simulink library "SUB_L4_Task_10ms_SUB_STATE_CONTROL"  (R2018a)
settings: Solver=VariableStepAuto  StartTime=0.0  StopTime=10.0  RelTol=1e-3
undefined symbols (not defined in the file or in its folder): ENUM_J1939_SWITCH_T, magnitude
libraries: EmE_MBD_Blockset x24, PTC_MBDS_LIB x5, simulink x5
settings Model: Creator=Chris.Balton  LastModifiedBy=Gavin.Coelho

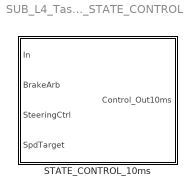
== system SUB_L4_Task_10ms_SUB_STATE_CONTROL ==
  STATE_CONTROL_10ms : Subsystem

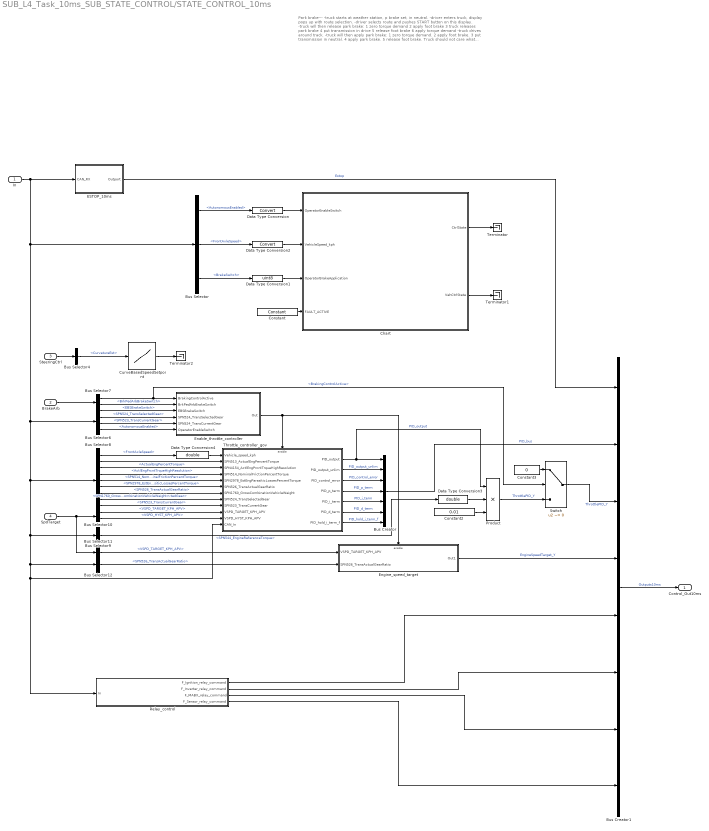
== system SUB_L4_Task_10ms_SUB_STATE_CONTROL/STATE_CONTROL_10ms ==
  note: Park brake---
      |
      |
      | -truck starts at weather station, p brake set, in neutral.
      | -driver enters truck, display pops up with route selection.
      | -driver selects route and pushes START button on this display.
      |
      | -truck will then release park brake:
      | 	1 zero torque demand
      | 	2 apply foot brake
      | 	3 truck releases park brake
      | 	4 put transmission in drive
      | 	5 release foot brake
      | 	6 apply torque demand
      |
      | -truck drives around track.
      |
      | -truck will then apply park brake:
      |
      | 	1 zero torque demand.
      | 	2 apply foot brake.
      | 	3 put transmission in neutral.
      | 	4 apply park brake.
      | 	5 release foot brake.
      |
      | Truck should not care what position the driver demanded transmission selector is in (stalk
      | position)
  In : Inport
  BrakeArb : Inport  Port=2
  SteeringCtrl : Inport  Port=3
  SpdTarget : Inport  Port=4
  Bus Creator : BusCreator  Inputs=7
  Bus Creator1 : BusCreator  Inputs=8
  Bus Selector : BusSelector  OutputSignals=DIO_Bus.AutonomousEnabled,CAN.EBC2_0B.FrontAxleSpeed,CAN.CCVS_31.BrakeSwitch
  Bus Selector10 : BusSelector  OutputSignals=VSPD_TARGET_KPH_APV,VSPD_HYST_KPH_APV
  Bus Selector11 : BusSelector  OutputSignals=VSPD_TARGET_KPH_APV
  Bus Selector12 : BusSelector  OutputSignals=CAN.ETC2_03.SPN526_TransActualGearRatio
  Bus Selector4 : BusSelector  OutputSignals=CurvatureEst
  Bus Selector6 : BusSelector  OutputSignals=CAN.EBC1_0B.EBSBrakeSwitch,CAN.ETC2_03.SPN524_TransSelectedGear,CAN.ETC2_03.SPN523_TransCurrentGear,AutonomousState.AutonomousEnabled
  Bus Selector7 : BusSelector  OutputSignals=BrakingControlActive,BrkPedArbBrakeSwitch
  Bus Selector8 : BusSelector  OutputSignals=CAN.EBC2_0B.FrontAxleSpeed,CAN.EEC1_00.ActualEngPercentTorque,CAN.EEC1_00.ActlEngPrcntTrqueHighResolution,CAN.EEC3_00.SPN514_NominalFrictionPercentTorque,CAN.EEC3_00.SPN2978_EstEngParasiticLossesPercentTorque,CAN.ETC2_03.SPN526_TransActualGearRatio,CAN.CVW_0B.SPN1760_GrossCombinationVehicleWeight,CAN.ETC2_03.SPN524_TransSelectedGear,CAN.ETC2_03.SPN523_TransCurrentGear
  Bus Selector9 : BusSelector  OutputSignals=CAN.EC1_00.SPN544_EngineReferenceTorque
  Chart : Stateflow chart  TreatAsAtomicUnit=on
      settings: CopyFcn=|
      | if strcmp(get(gcbh, 'LinkStatus'), 'resolved')
      |     set(gcbh, 'LinkStatus', 'none');
      | end
  Constant : PTC_MBDS_LIB/Extras/Sources/Constant  Value2=false  PTC_MBDS_BlockVersion=5.41  PTC_BlockType=PTC_MBDS_Constant
      settings: SourceProductName=PACCAR Technical Center MBDS Library
  Constant2 : Constant  Value=0.01
  Constant3 : Constant  Value=0
  CurveBasedSpeedSetpoint : Lookup_n-D  NumberOfTableDimensions=1  BreakpointsForDimension1=[-.25,-.1 0 .1 .25]  Table=[25 30 35 30 25]  ExtrapMethod=Clip  UseLastTableValue=on  InputSameDT=on
      settings: AttributesFormatString=|
      | X: %<BreakpointsForDimension1>
      | Y: %<Table>
  Data Type Conversion4 : DataTypeConversion  OutDataTypeStr=double  SaturateOnIntegerOverflow=on
  Data Type Conversion : DataTypeConversion
  Data Type Conversion1 : DataTypeConversion  OutDataTypeStr=uint8
  Data Type Conversion2 : DataTypeConversion
  Data Type Conversion3 : DataTypeConversion  OutDataTypeStr=double
  ESTOP_10ms : Subsystem
  Enable_throttle_controller : Subsystem
  Engine_speed_target : Subsystem  TreatAsAtomicUnit=on
  Product : Product  Inputs=3  InputSameDT=on
  Relay_control : Subsystem
  Switch : Switch  Criteria=u2 ~= 0
  Terminator : Terminator
      settings: InitFcn=|
      | try
      |    MBDS_BlockCallback('Update', gcb);
      | end
  Terminator1 : Terminator
      settings: InitFcn=|
      | try
      |    MBDS_BlockCallback('Update', gcb);
      | end
  Terminator2 : Terminator
      settings: InitFcn=|
      | try
      |    MBDS_BlockCallback('Update', gcb);
      | end
  Throttle_controller_gov : Subsystem  TreatAsAtomicUnit=on
  Control_Out10ms : Outport
  wires:
  Relay_control/4(F_Sensor_relay_command) -> Bus Creator1/8
  Relay_control/1(F_Ignition_relay_command) -> Bus Creator1/5
  Relay_control/3(F_MABX_relay_command) -> Bus Creator1/7
  Relay_control/2(F_Inverter_relay_command) -> Bus Creator1/6
  Data Type Conversion3/1 -> Product/2
  Bus Selector12/1 -> Engine_speed_target/2(SPN526_TransActualGearRatio)  "<SPN526_TransActualGearRatio>"
  Engine_speed_target/1(Out1) -> Bus Creator1/4  "EngineSpeedTarget_Y"
  Bus Selector11/1 -> Engine_speed_target/1(VSPD_TARGET_KPH_APV)  "<VSPD_TARGET_KPH_APV>"
  Bus Selector/1 -> Data Type Conversion/1  "<AutonomousEnabled>"
  Bus Selector/2 -> Data Type Conversion2/1  "<FrontAxleSpeed>"
  Bus Selector/3 -> Data Type Conversion1/1  "<BrakeSwitch>"
  Chart/1(CtrlState) -> Terminator/1
  Chart/2(VehCtrlState) -> Terminator1/1
  Bus Creator1/1 -> Control_Out10ms/1  "Outputs10ms"
  ESTOP_10ms/1(Outport) -> Bus Creator1/1  "Estop"
  Data Type Conversion/1 -> Chart/1(OperatorEnableSwitch)
  BrakeArb/1 -> Bus Selector7/1
  SteeringCtrl/1 -> Bus Selector4/1
  Bus Selector4/1 -> CurveBasedSpeedSetpoint/1  "<CurvatureEst>"
  Data Type Conversion1/1 -> Chart/3(OperatorBrakeApplication)
  Data Type Conversion2/1 -> Chart/2(VehicleSpeed_kph)
  Switch/1 -> Bus Creator1/3  "ThrottlePID_Y"
  Bus Selector6/4 -> Enable_throttle_controller/6(OperatorEnableSwitch)  "<AutonomousEnabled>"
  Bus Selector6/3 -> Enable_throttle_controller/5(SPN524_TransCurrentGear)  "<SPN523_TransCurrentGear>"
  Bus Selector6/2 -> Enable_throttle_controller/4(SPN524_TransSelectedGear)  "<SPN524_TransSelectedGear>"
  Bus Selector6/1 -> Enable_throttle_controller/3(EBSBrakeSwitch)  "<EBSBrakeSwitch>"
  Bus Selector7/2 -> Enable_throttle_controller/2(BrkPedArbBrakeSwitch)  "<BrkPedArbBrakeSwitch>"
  Bus Selector7/1 -> Switch/2, Enable_throttle_controller/1(BrakingControlActive)  "<BrakingControlActive>"
  Enable_throttle_controller/1(Out) -> Engine_speed_target/Enable, Throttle_controller_gov/Enable
  Bus Selector8/1 -> Data Type Conversion4/1  "<FrontAxleSpeed>"
  Bus Selector8/9 -> Throttle_controller_gov/9(SPN523_TransCurrentGear)  "<SPN523_TransCurrentGear>"
  Bus Selector8/8 -> Throttle_controller_gov/8(SPN524_TransSelectedGear)  "<SPN524_TransSelectedGear>"
  Bus Selector8/2 -> Throttle_controller_gov/2(SPN513_ActualEngPercentTorque)  "<ActualEngPercentTorque>"
  Bus Selector8/3 -> Throttle_controller_gov/3(SPN4154_ActlEngPrcntTrqueHighResolution)  "<ActlEngPrcntTrqueHighResolution>"
  Bus Selector8/4 -> Throttle_controller_gov/4(SPN514_NominalFrictionPercentTorque)  "<SPN514_NominalFrictionPercentTorque>"
  Bus Selector8/5 -> Throttle_controller_gov/5(SPN2978_EstEngParasiticLossesPercentTorque)  "<SPN2978_EstEngParasiticLossesPercentTorque>"
  Bus Selector8/6 -> Throttle_controller_gov/6(SPN526_TransActualGearRatio)  "<SPN526_TransActualGearRatio>"
  Bus Selector8/7 -> Throttle_controller_gov/7(SPN1760_GrossCombinationVehicleWeight)  "<SPN1760_GrossCombinationVehicleWeight>"
  In/1 -> ESTOP_10ms/1(CAN_RX), Bus Selector/1, Throttle_controller_gov/12(CAN_In), Relay_control/1(In), Bus Selector12/1, Bus Selector9/1, Bus Selector8/1, Bus Selector6/1
  Bus Selector9/1 -> Data Type Conversion3/1  "<SPN544_EngineReferenceTorque>"
  Constant2/1 -> Product/3
  SpdTarget/1 -> Bus Selector10/1, Bus Selector11/1
  Bus Selector10/2 -> Throttle_controller_gov/11(VSPD_HYST_KPH_APV)  "<VSPD_HYST_KPH_APV>"
  Bus Selector10/1 -> Throttle_controller_gov/10(VSPD_TARGET_KPH_APV)  "<VSPD_TARGET_KPH_APV>"
  Data Type Conversion4/1 -> Throttle_controller_gov/1(Vehicle_speed_kph)
  CurveBasedSpeedSetpoint/1 -> Terminator2/1
  Throttle_controller_gov/1(PID_output) -> Product/1, Bus Creator/1  "PID_output"
  Throttle_controller_gov/7(PID_hold_i_term_f) -> Bus Creator/7  "PID_hold_i_term_f"
  Throttle_controller_gov/6(PID_d_term) -> Bus Creator/6  "PID_d_term"
  Throttle_controller_gov/5(PID_i_term) -> Bus Creator/5  "PID_i_term"
  Throttle_controller_gov/4(PID_p_term) -> Bus Creator/4  "PID_p_term"
  Throttle_controller_gov/3(PID_control_error) -> Bus Creator/3  "PID_control_error"
  Throttle_controller_gov/2(PID_output_unlim) -> Bus Creator/2  "PID_output_unlim"
  Bus Creator/1 -> Bus Creator1/2  "PID_bus"
  Product/1 -> Switch/3  "ThrottlePID_Y"
  Constant3/1 -> Switch/1
  Constant/1 -> Chart/4(FAULT_ACTIVE)

== system SUB_L4_Task_10ms_SUB_STATE_CONTROL/STATE_CONTROL_10ms/ESTOP_10ms ==
  CAN_RX : Inport
  Bus Creator : BusCreator  Inputs=1
  Constant : PTC_MBDS_LIB/Extras/Sources/Constant  Value2=false  PTC_MBDS_BlockVersion=5.41  PTC_BlockType=PTC_MBDS_Constant
      settings: SourceProductName=PACCAR Technical Center MBDS Library
  Terminator1 : Terminator
  Outport : Outport
  wires:
  Constant/1 -> Bus Creator/1
  CAN_RX/1 -> Terminator1/1
  Bus Creator/1 -> Outport/1  "Estop"

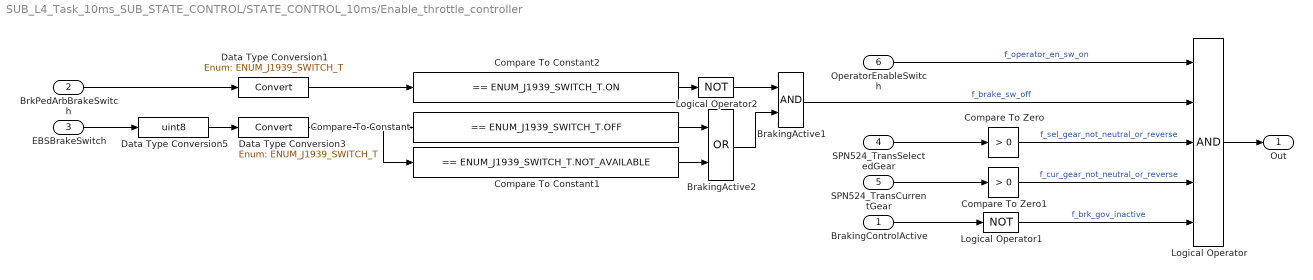
== system SUB_L4_Task_10ms_SUB_STATE_CONTROL/STATE_CONTROL_10ms/Enable_throttle_controller ==
  BrakingControlActive : Inport
  BrkPedArbBrakeSwitch : Inport  Port=2
  EBSBrakeSwitch : Inport  Port=3
  SPN524_TransSelectedGear : Inport  Port=4
  SPN524_TransCurrentGear : Inport  Port=5
  OperatorEnableSwitch : Inport  Port=6
  BrakingActive1 : Logic  OutDataTypeStr=boolean
  BrakingActive2 : Logic  Operator=OR  OutDataTypeStr=boolean
  Compare To Constant : simulink/Logic and Bit Operations/Compare To Constant  relop===  const=ENUM_J1939_SWITCH_T.OFF  OutDataTypeStr=boolean
  Compare To Constant1 : simulink/Logic and Bit Operations/Compare To Constant  relop===  const=ENUM_J1939_SWITCH_T.NOT_AVAILABLE  OutDataTypeStr=boolean
  Compare To Constant2 : simulink/Logic and Bit Operations/Compare To Constant  relop===  const=ENUM_J1939_SWITCH_T.ON  OutDataTypeStr=boolean
  Compare To Zero : simulink/Logic and Bit Operations/Compare To Zero  relop=>  OutDataTypeStr=boolean
  Compare To Zero1 : simulink/Logic and Bit Operations/Compare To Zero  relop=>  OutDataTypeStr=boolean
  Data Type Conversion1 : DataTypeConversion  OutDataTypeStr=Enum: ENUM_J1939_SWITCH_T
      settings: AttributesFormatString=%<OutDataTypeStr>
  Data Type Conversion3 : DataTypeConversion  OutDataTypeStr=Enum: ENUM_J1939_SWITCH_T
      settings: AttributesFormatString=%<OutDataTypeStr>
  Data Type Conversion5 : DataTypeConversion  OutDataTypeStr=uint8
      settings: AttributesFormatString=%<OutDataTypeStr>
  Logical Operator : Logic  Inputs=5  OutDataTypeStr=boolean
  Logical Operator1 : Logic  Operator=NOT  Inputs=4  OutDataTypeStr=boolean
  Logical Operator2 : Logic  Operator=NOT  Inputs=4  OutDataTypeStr=boolean
  Out : Outport
  wires:
  SPN524_TransSelectedGear/1 -> Compare To Zero/1
  SPN524_TransCurrentGear/1 -> Compare To Zero1/1
  BrakingControlActive/1 -> Logical Operator1/1
  Logical Operator1/1 -> Logical Operator/5  "f_brk_gov_inactive"
  Compare To Zero1/1 -> Logical Operator/4  "f_cur_gear_not_neutral_or_reverse"
  Compare To Zero/1 -> Logical Operator/3  "f_sel_gear_not_neutral_or_reverse"
  Logical Operator/1 -> Out/1
  OperatorEnableSwitch/1 -> Logical Operator/1  "f_operator_en_sw_on"
  BrakingActive1/1 -> Logical Operator/2  "f_brake_sw_off"
  EBSBrakeSwitch/1 -> Data Type Conversion5/1
  BrkPedArbBrakeSwitch/1 -> Data Type Conversion1/1
  Logical Operator2/1 -> BrakingActive1/1
  Compare To Constant/1 -> BrakingActive2/1
  Compare To Constant1/1 -> BrakingActive2/2
  BrakingActive2/1 -> BrakingActive1/2
  Data Type Conversion3/1 -> Compare To Constant/1, Compare To Constant1/1
  Data Type Conversion1/1 -> Compare To Constant2/1
  Compare To Constant2/1 -> Logical Operator2/1
  Data Type Conversion5/1 -> Data Type Conversion3/1

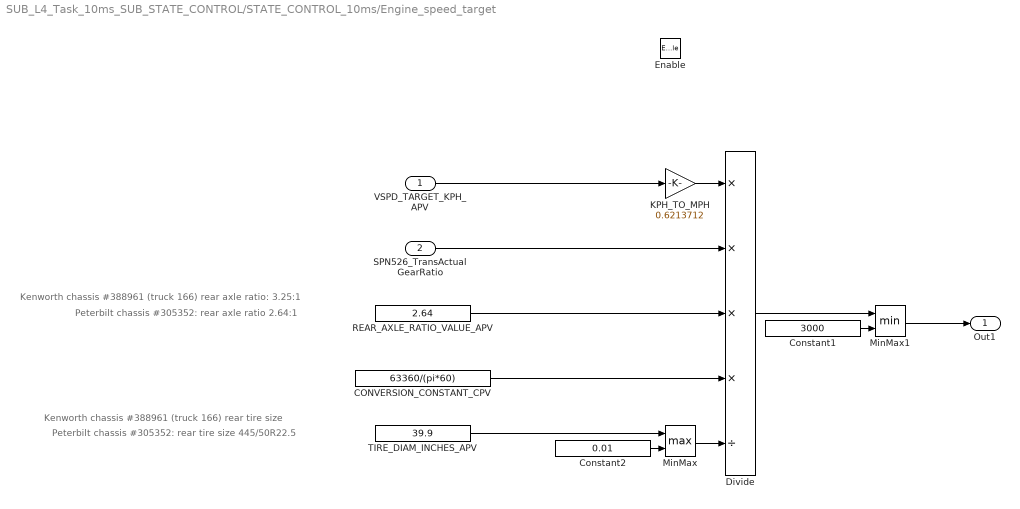
== system SUB_L4_Task_10ms_SUB_STATE_CONTROL/STATE_CONTROL_10ms/Engine_speed_target ==
  note: Kenworth chassis #388961 (truck 166) rear tire size
  note: Kenworth chassis #388961 (truck 166) rear axle ratio: 3.25:1
  note: Peterbilt chassis #305352: rear axle ratio 2.64:1
  note: Peterbilt chassis #305352: rear tire size 445/50R22.5
  VSPD_TARGET_KPH_APV : Inport
  SPN526_TransActualGearRatio : Inport  Port=2
  Enable : EnablePort  StatesWhenEnabling=reset
  CONVERSION_CONSTANT_CPV : Constant  Value=63360/(pi*60)
  Constant1 : Constant  Value=3000
  Constant2 : Constant  Value=0.01
  Divide : Product  Inputs=****/  InputSameDT=on
  KPH_TO_MPH : Gain  Gain=0.6213712  OutDataTypeStr=double
  MinMax : MinMax  Function=max  Inputs=2  InputSameDT=on
  MinMax1 : MinMax  Inputs=2  InputSameDT=on
  REAR_AXLE_RATIO_VALUE_APV : Constant  Value=2.64
  TIRE_DIAM_INCHES_APV : Constant  Value=39.9
  Out1 : Outport  OutputWhenDisabled=reset  InitialOutput=0
  wires:
  KPH_TO_MPH/1 -> Divide/1
  Constant1/1 -> MinMax1/2
  MinMax1/1 -> Out1/1
  Constant2/1 -> MinMax/2
  MinMax/1 -> Divide/5
  SPN526_TransActualGearRatio/1 -> Divide/2
  VSPD_TARGET_KPH_APV/1 -> KPH_TO_MPH/1
  REAR_AXLE_RATIO_VALUE_APV/1 -> Divide/3
  TIRE_DIAM_INCHES_APV/1 -> MinMax/1
  CONVERSION_CONSTANT_CPV/1 -> Divide/4
  Divide/1 -> MinMax1/1

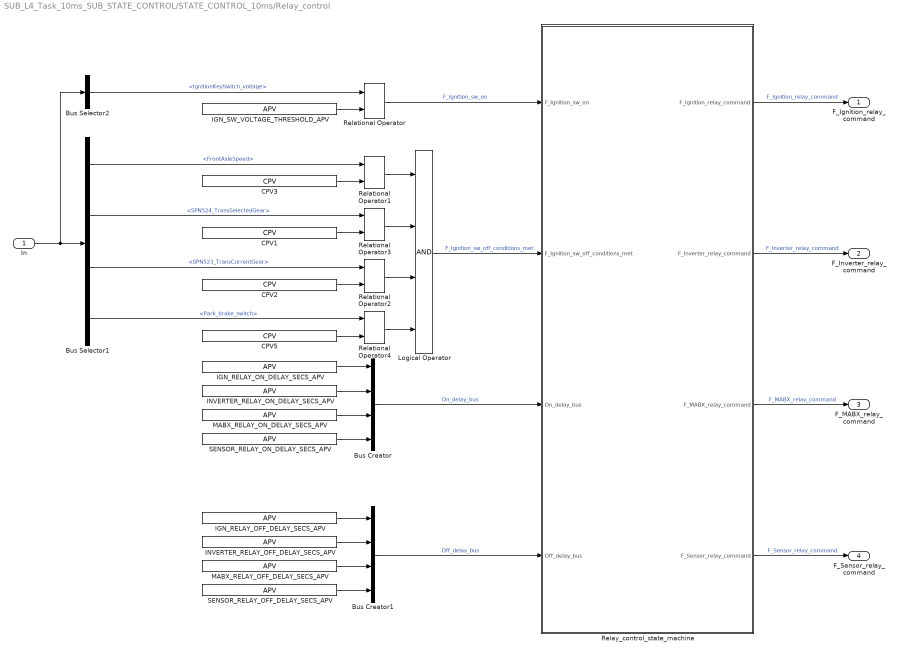
== system SUB_L4_Task_10ms_SUB_STATE_CONTROL/STATE_CONTROL_10ms/Relay_control ==
  In : Inport
  Bus Creator : BusCreator  Inputs=4
  Bus Creator1 : BusCreator  Inputs=4
  Bus Selector1 : BusSelector  OutputSignals=CAN.EBC2_0B.FrontAxleSpeed,CAN.ETC2_03.SPN524_TransSelectedGear,CAN.ETC2_03.SPN523_TransCurrentGear,CAN.CCVS_31.Park_brake_switch
  Bus Selector2 : BusSelector  OutputSignals=DIO_Bus.IgnitionKeySwitch_voltage
  CPV1 : EmE_MBD_Blockset/Sources/CPV  conval=0
      settings: SourceProductName=PACCAR EmE MBD Blockset
  CPV2 : EmE_MBD_Blockset/Sources/CPV  conval=0
      settings: SourceProductName=PACCAR EmE MBD Blockset
  CPV3 : EmE_MBD_Blockset/Sources/CPV  conval=0
      settings: SourceProductName=PACCAR EmE MBD Blockset
  CPV5 : EmE_MBD_Blockset/Sources/CPV  conval=1
      settings: SourceProductName=PACCAR EmE MBD Blockset
  IGN_RELAY_OFF_DELAY_SECS_APV : EmE_MBD_Blockset/Sources/APV  conval=0.2
      settings: SourceProductName=PACCAR EmE MBD Blockset
  IGN_RELAY_ON_DELAY_SECS_APV : EmE_MBD_Blockset/Sources/APV  conval=0.2
      settings: SourceProductName=PACCAR EmE MBD Blockset
  IGN_SW_VOLTAGE_THRESHOLD_APV : EmE_MBD_Blockset/Sources/APV  conval=6
      settings: SourceProductName=PACCAR EmE MBD Blockset
  INVERTER_RELAY_OFF_DELAY_SECS_APV : EmE_MBD_Blockset/Sources/APV  conval=0
      settings: SourceProductName=PACCAR EmE MBD Blockset
  INVERTER_RELAY_ON_DELAY_SECS_APV : EmE_MBD_Blockset/Sources/APV  conval=0
      settings: SourceProductName=PACCAR EmE MBD Blockset
  Logical Operator : Logic  Inputs=4  OutDataTypeStr=boolean
  MABX_RELAY_OFF_DELAY_SECS_APV : EmE_MBD_Blockset/Sources/APV  conval=0
      settings: SourceProductName=PACCAR EmE MBD Blockset
  MABX_RELAY_ON_DELAY_SECS_APV : EmE_MBD_Blockset/Sources/APV  conval=0
      settings: SourceProductName=PACCAR EmE MBD Blockset
  Relational Operator : EmE_MBD_Blockset/Logic and Bit Operations/Relational Operator  func=>=
      settings: SourceProductName=PACCAR EmE MBD Blockset
  Relational Operator1 : EmE_MBD_Blockset/Logic and Bit Operations/Relational Operator  func=<=
      settings: SourceProductName=PACCAR EmE MBD Blockset
  Relational Operator2 : EmE_MBD_Blockset/Logic and Bit Operations/Relational Operator  func===
      settings: SourceProductName=PACCAR EmE MBD Blockset
  Relational Operator3 : EmE_MBD_Blockset/Logic and Bit Operations/Relational Operator  func===
      settings: SourceProductName=PACCAR EmE MBD Blockset
  Relational Operator4 : EmE_MBD_Blockset/Logic and Bit Operations/Relational Operator  func===
      settings: SourceProductName=PACCAR EmE MBD Blockset
  Relay_control_state_machine : Stateflow chart  TreatAsAtomicUnit=on
  SENSOR_RELAY_OFF_DELAY_SECS_APV : EmE_MBD_Blockset/Sources/APV  conval=0
      settings: SourceProductName=PACCAR EmE MBD Blockset
  SENSOR_RELAY_ON_DELAY_SECS_APV : EmE_MBD_Blockset/Sources/APV  conval=0
      settings: SourceProductName=PACCAR EmE MBD Blockset
  F_Ignition_relay_command : Outport
  F_Inverter_relay_command : Outport  Port=2
  F_MABX_relay_command : Outport  Port=3
  F_Sensor_relay_command : Outport  Port=4
  wires:
  Bus Selector1/1 -> Relational Operator1/1  "<FrontAxleSpeed>"
  Relay_control_state_machine/2(F_Inverter_relay_command) -> F_Inverter_relay_command/1  "F_Inverter_relay_command"
  Bus Selector1/3 -> Relational Operator2/1  "<SPN523_TransCurrentGear>"
  IGN_RELAY_ON_DELAY_SECS_APV/1 -> Bus Creator/1
  Bus Selector2/1 -> Relational Operator/1  "<IgnitionKeySwitch_voltage>"
  Bus Selector1/2 -> Relational Operator3/1  "<SPN524_TransSelectedGear>"
  Relay_control_state_machine/1(F_Ignition_relay_command) -> F_Ignition_relay_command/1  "F_Ignition_relay_command"
  Bus Selector1/4 -> Relational Operator4/1  "<Park_brake_switch>"
  Relay_control_state_machine/3(F_MABX_relay_command) -> F_MABX_relay_command/1  "F_MABX_relay_command"
  Relay_control_state_machine/4(F_Sensor_relay_command) -> F_Sensor_relay_command/1  "F_Sensor_relay_command"
  Relational Operator3/1 -> Logical Operator/2
  CPV2/1 -> Relational Operator2/2
  Relational Operator2/1 -> Logical Operator/3
  CPV1/1 -> Relational Operator3/2
  Relational Operator/1 -> Relay_control_state_machine/1(F_Ignition_sw_on)  "F_Ignition_sw_on"
  CPV3/1 -> Relational Operator1/2
  Relational Operator4/1 -> Logical Operator/4
  Relational Operator1/1 -> Logical Operator/1
  Bus Creator1/1 -> Relay_control_state_machine/4(Off_delay_bus)  "Off_delay_bus"
  INVERTER_RELAY_ON_DELAY_SECS_APV/1 -> Bus Creator/2
  Logical Operator/1 -> Relay_control_state_machine/2(F_Ignition_sw_off_conditions_met)  "F_Ignition_sw_off_conditions_met"
  SENSOR_RELAY_ON_DELAY_SECS_APV/1 -> Bus Creator/4
  MABX_RELAY_ON_DELAY_SECS_APV/1 -> Bus Creator/3
  Bus Creator/1 -> Relay_control_state_machine/3(On_delay_bus)  "On_delay_bus"
  CPV5/1 -> Relational Operator4/2
  MABX_RELAY_OFF_DELAY_SECS_APV/1 -> Bus Creator1/3
  SENSOR_RELAY_OFF_DELAY_SECS_APV/1 -> Bus Creator1/4
  IGN_RELAY_OFF_DELAY_SECS_APV/1 -> Bus Creator1/1
  IGN_SW_VOLTAGE_THRESHOLD_APV/1 -> Relational Operator/2
  INVERTER_RELAY_OFF_DELAY_SECS_APV/1 -> Bus Creator1/2
  In/1 -> Bus Selector1/1, Bus Selector2/1

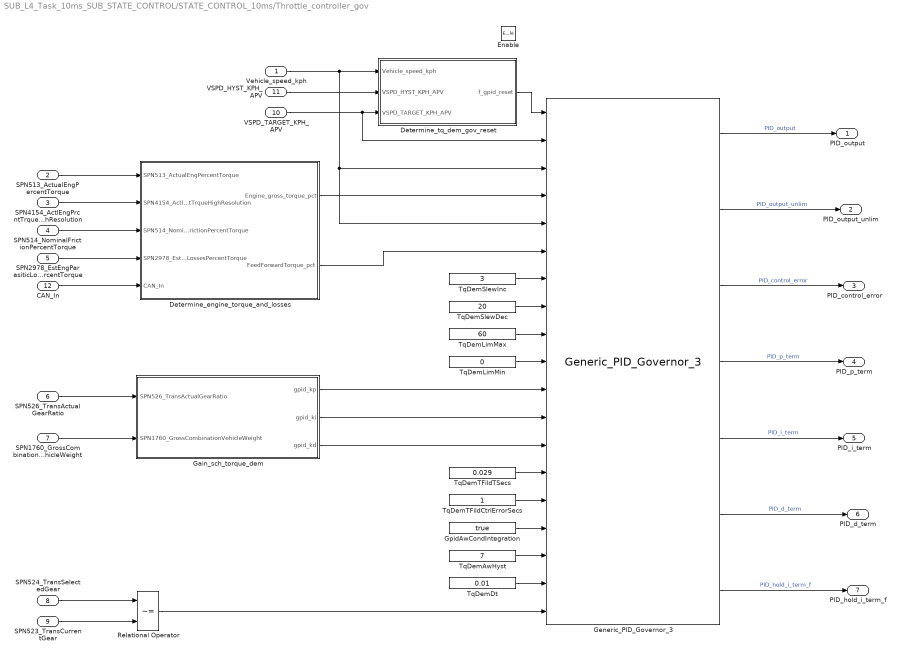
== system SUB_L4_Task_10ms_SUB_STATE_CONTROL/STATE_CONTROL_10ms/Throttle_controller_gov ==
  Vehicle_speed_kph : Inport
  SPN513_ActualEngPercentTorque : Inport  Port=2
  SPN4154_ActlEngPrcntTrqueHighResolution : Inport  Port=3
  SPN514_NominalFrictionPercentTorque : Inport  Port=4
  SPN2978_EstEngParasiticLossesPercentTorque : Inport  Port=5
  SPN526_TransActualGearRatio : Inport  Port=6
  SPN1760_GrossCombinationVehicleWeight : Inport  Port=7
  SPN524_TransSelectedGear : Inport  Port=8
  SPN523_TransCurrentGear : Inport  Port=9
  VSPD_TARGET_KPH_APV : Inport  Port=10
  VSPD_HYST_KPH_APV : Inport  Port=11
  CAN_In : Inport  Port=12
  Enable : EnablePort  StatesWhenEnabling=reset
  Determine_engine_torque_and_losses : Subsystem
  Determine_tq_dem_gov_reset : Subsystem
  Gain_sch_torque_dem : Subsystem
  Generic_PID_Governor_3 : EmE_MBD_Blockset/Controllers/Generic_PID_Governor_3
      settings: SourceProductName=PACCAR EmE MBD Blockset
  GpidAwCondIntegration : Constant  Value=true
  Relational Operator : RelationalOperator  Operator=~=  OutDataTypeStr=boolean  RndMeth=Nearest  InputSameDT=on
  TqDemAwHyst : Constant  Value=7
  TqDemDt : Constant  Value=0.01
  TqDemLimMax : Constant  Value=60
  TqDemLimMin : Constant  Value=0
  TqDemSlewDec : Constant  Value=20
  TqDemSlewInc : Constant  Value=3
  TqDemTFildCtrlErrorSecs : Constant
  TqDemTFildTSecs : Constant  Value=0.029
  PID_output : Outport  OutputWhenDisabled=reset  InitialOutput=0
  PID_output_unlim : Outport  Port=2  OutputWhenDisabled=reset  InitialOutput=0
  PID_control_error : Outport  Port=3  OutputWhenDisabled=reset  InitialOutput=0
  PID_p_term : Outport  Port=4  OutputWhenDisabled=reset  InitialOutput=0
  PID_i_term : Outport  Port=5  OutputWhenDisabled=reset  InitialOutput=0
  PID_d_term : Outport  Port=6  OutputWhenDisabled=reset  InitialOutput=0
  PID_hold_i_term_f : Outport  Port=7  OutputWhenDisabled=reset  InitialOutput=false
  wires:
  Vehicle_speed_kph/1 -> Generic_PID_Governor_3/5, Generic_PID_Governor_3/3, Determine_tq_dem_gov_reset/1(Vehicle_speed_kph)
  VSPD_HYST_KPH_APV/1 -> Determine_tq_dem_gov_reset/2(VSPD_HYST_KPH_APV)
  SPN513_ActualEngPercentTorque/1 -> Determine_engine_torque_and_losses/1(SPN513_ActualEngPercentTorque)
  SPN4154_ActlEngPrcntTrqueHighResolution/1 -> Determine_engine_torque_and_losses/2(SPN4154_ActlEngPrcntTrqueHighResolution)
  SPN514_NominalFrictionPercentTorque/1 -> Determine_engine_torque_and_losses/3(SPN514_NominalFrictionPercentTorque)
  SPN2978_EstEngParasiticLossesPercentTorque/1 -> Determine_engine_torque_and_losses/4(SPN2978_EstEngParasiticLossesPercentTorque)
  SPN526_TransActualGearRatio/1 -> Gain_sch_torque_dem/1(SPN526_TransActualGearRatio)
  SPN1760_GrossCombinationVehicleWeight/1 -> Gain_sch_torque_dem/2(SPN1760_GrossCombinationVehicleWeight)
  SPN523_TransCurrentGear/1 -> Relational Operator/2
  SPN524_TransSelectedGear/1 -> Relational Operator/1
  Determine_tq_dem_gov_reset/1(f_gpid_reset) -> Generic_PID_Governor_3/1
  Determine_engine_torque_and_losses/1(Engine_gross_torque_pct) -> Generic_PID_Governor_3/4
  Determine_engine_torque_and_losses/2(FeedForwardTorque_pct) -> Generic_PID_Governor_3/6
  Relational Operator/1 -> Generic_PID_Governor_3/19
  Gain_sch_torque_dem/1(gpid_kp) -> Generic_PID_Governor_3/11
  Gain_sch_torque_dem/2(gpid_ki) -> Generic_PID_Governor_3/12
  Gain_sch_torque_dem/3(gpid_kd) -> Generic_PID_Governor_3/13
  TqDemLimMin/1 -> Generic_PID_Governor_3/10
  TqDemLimMax/1 -> Generic_PID_Governor_3/9
  TqDemSlewInc/1 -> Generic_PID_Governor_3/7
  TqDemSlewDec/1 -> Generic_PID_Governor_3/8
  TqDemTFildTSecs/1 -> Generic_PID_Governor_3/14
  TqDemTFildCtrlErrorSecs/1 -> Generic_PID_Governor_3/15
  GpidAwCondIntegration/1 -> Generic_PID_Governor_3/16
  TqDemAwHyst/1 -> Generic_PID_Governor_3/17
  TqDemDt/1 -> Generic_PID_Governor_3/18
  Generic_PID_Governor_3/2 -> PID_output_unlim/1  "PID_output_unlim"
  Generic_PID_Governor_3/1 -> PID_output/1  "PID_output"
  Generic_PID_Governor_3/3 -> PID_control_error/1  "PID_control_error"
  Generic_PID_Governor_3/4 -> PID_p_term/1  "PID_p_term"
  Generic_PID_Governor_3/5 -> PID_i_term/1  "PID_i_term"
  Generic_PID_Governor_3/6 -> PID_d_term/1  "PID_d_term"
  Generic_PID_Governor_3/7 -> PID_hold_i_term_f/1  "PID_hold_i_term_f"
  VSPD_TARGET_KPH_APV/1 -> Generic_PID_Governor_3/2, Determine_tq_dem_gov_reset/3(VSPD_TARGET_KPH_APV)
  CAN_In/1 -> Determine_engine_torque_and_losses/5(CAN_In)

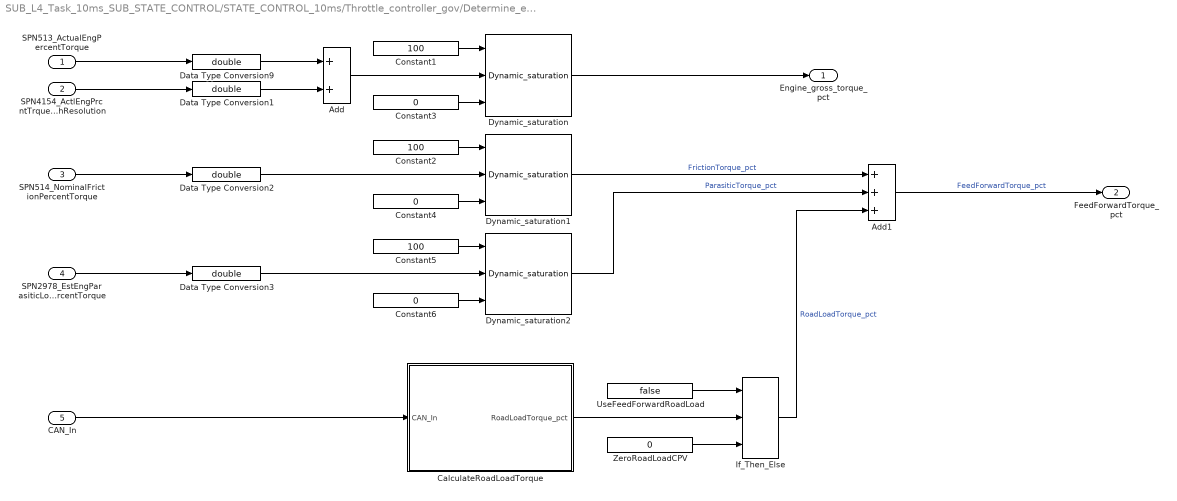
== system SUB_L4_Task_10ms_SUB_STATE_CONTROL/STATE_CONTROL_10ms/Throttle_controller_gov/Determine_engine_torque_and_losses ==
  SPN513_ActualEngPercentTorque : Inport
  SPN4154_ActlEngPrcntTrqueHighResolution : Inport  Port=2
  SPN514_NominalFrictionPercentTorque : Inport  Port=3
  SPN2978_EstEngParasiticLossesPercentTorque : Inport  Port=4
  CAN_In : Inport  Port=5
  Add : Sum  InputSameDT=on
  Add1 : Sum  Inputs=+++  InputSameDT=on
  CalculateRoadLoadTorque : Subsystem
  Constant1 : Constant  Value=100
  Constant2 : Constant  Value=100
  Constant3 : Constant  Value=0
  Constant4 : Constant  Value=0
  Constant5 : Constant  Value=100
  Constant6 : Constant  Value=0
  Data Type Conversion{1..3,9} (4 alike) : DataTypeConversion  OutDataTypeStr=double  SaturateOnIntegerOverflow=on
  Dynamic_saturation : EmE_MBD_Blockset/Discontinuities/Dynamic_saturation
      settings: SourceProductName=PACCAR EmE MBD Blockset
  Dynamic_saturation1 : EmE_MBD_Blockset/Discontinuities/Dynamic_saturation
      settings: SourceProductName=PACCAR EmE MBD Blockset
  Dynamic_saturation2 : EmE_MBD_Blockset/Discontinuities/Dynamic_saturation
      settings: SourceProductName=PACCAR EmE MBD Blockset
  If_Then_Else : EmE_MBD_Blockset/Signal Routing/If_Then_Else
      settings: SourceProductName=PACCAR EmE MBD Blockset
  UseFeedForwardRoadLoad : Constant  Value=false  OutDataTypeStr=boolean
  ZeroRoadLoadCPV : Constant  Value=0
  Engine_gross_torque_pct : Outport
  FeedForwardTorque_pct : Outport  Port=2
  wires:
  SPN513_ActualEngPercentTorque/1 -> Data Type Conversion9/1
  SPN4154_ActlEngPrcntTrqueHighResolution/1 -> Data Type Conversion1/1
  Add/1 -> Dynamic_saturation/2
  Constant3/1 -> Dynamic_saturation/3
  Constant1/1 -> Dynamic_saturation/1
  SPN514_NominalFrictionPercentTorque/1 -> Data Type Conversion2/1
  Constant4/1 -> Dynamic_saturation1/3
  Constant2/1 -> Dynamic_saturation1/1
  SPN2978_EstEngParasiticLossesPercentTorque/1 -> Data Type Conversion3/1
  Constant6/1 -> Dynamic_saturation2/3
  Constant5/1 -> Dynamic_saturation2/1
  Dynamic_saturation1/1 -> Add1/1  "FrictionTorque_pct"
  Dynamic_saturation2/1 -> Add1/2  "ParasiticTorque_pct"
  Dynamic_saturation/1 -> Engine_gross_torque_pct/1
  Add1/1 -> FeedForwardTorque_pct/1  "FeedForwardTorque_pct"
  Data Type Conversion9/1 -> Add/1
  Data Type Conversion1/1 -> Add/2
  Data Type Conversion2/1 -> Dynamic_saturation1/2
  Data Type Conversion3/1 -> Dynamic_saturation2/2
  CAN_In/1 -> CalculateRoadLoadTorque/1(CAN_In)
  CalculateRoadLoadTorque/1(RoadLoadTorque_pct) -> If_Then_Else/2
  If_Then_Else/1 -> Add1/3  "RoadLoadTorque_pct"
  ZeroRoadLoadCPV/1 -> If_Then_Else/3
  UseFeedForwardRoadLoad/1 -> If_Then_Else/1

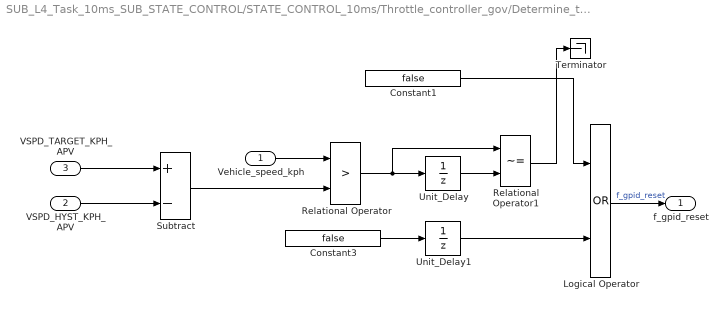
== system SUB_L4_Task_10ms_SUB_STATE_CONTROL/STATE_CONTROL_10ms/Throttle_controller_gov/Determine_tq_dem_gov_reset ==
  Vehicle_speed_kph : Inport
  VSPD_HYST_KPH_APV : Inport  Port=2
  VSPD_TARGET_KPH_APV : Inport  Port=3
  Constant1 : Constant  Value=false
  Constant3 : Constant  Value=false
  Logical Operator : Logic  Operator=OR  AllPortsSameDT=off  OutDataTypeStr=boolean
  Relational Operator : RelationalOperator  Operator=>  OutDataTypeStr=boolean  RndMeth=Nearest  InputSameDT=on
  Relational Operator1 : RelationalOperator  Operator=~=  OutDataTypeStr=boolean  RndMeth=Nearest  InputSameDT=on
  Subtract : Sum  Inputs=+-  InputSameDT=on
  Terminator : Terminator
  Unit_Delay : UnitDelay  SampleTime=-1
      settings: AttributesFormatString=IC: %<vinit>
  Unit_Delay1 : UnitDelay  InitialCondition=true  SampleTime=-1
      settings: AttributesFormatString=IC: %<vinit>
  f_gpid_reset : Outport
  wires:
  VSPD_TARGET_KPH_APV/1 -> Subtract/1
  VSPD_HYST_KPH_APV/1 -> Subtract/2
  Vehicle_speed_kph/1 -> Relational Operator/1
  Subtract/1 -> Relational Operator/2
  Relational Operator/1 -> Unit_Delay/1, Relational Operator1/1
  Unit_Delay/1 -> Relational Operator1/2
  Relational Operator1/1 -> Terminator/1
  Logical Operator/1 -> f_gpid_reset/1  "f_gpid_reset"
  Unit_Delay1/1 -> Logical Operator/2
  Constant3/1 -> Unit_Delay1/1
  Constant1/1 -> Logical Operator/1

== system SUB_L4_Task_10ms_SUB_STATE_CONTROL/STATE_CONTROL_10ms/Throttle_controller_gov/Gain_sch_torque_dem ==
  SPN526_TransActualGearRatio : Inport
  SPN1760_GrossCombinationVehicleWeight : Inport  Port=2
  2D_Lookup_Table : PTC_MBDS_LIB/Extras/Lookup Tables/2D_Lookup_Table  ParameterObjectName=TQ_DEM_KP_DATA_MPV  InterpolationMethod=Linear  PTC_MBDS_BlockVersion=5.41  PTC_BlockType=PTC_MBDS_2D_Lookup_Table
      settings: SourceProductName=PACCAR Technical Center MBDS Library
      settings: AttributesFormatString=|
      | Row Axis: TQ_DEM_MASS_STEP_MPV (kg)
      | Column Axis: TQ_DEM_GEAR_RATIO_STEP_MPV (1)
      | Data Axis: TQ_DEM_KP_DATA_MPV (1)
      | Interpolation Method: Linear
  2D_Lookup_Table1 : PTC_MBDS_LIB/Extras/Lookup Tables/2D_Lookup_Table  ParameterObjectName=TQ_DEM_KI_DATA_MPV  InterpolationMethod=Linear  PTC_MBDS_BlockVersion=5.41  PTC_BlockType=PTC_MBDS_2D_Lookup_Table
      settings: SourceProductName=PACCAR Technical Center MBDS Library
      settings: AttributesFormatString=|
      | Row Axis: TQ_DEM_MASS_STEP_MPV (kg)
      | Column Axis: TQ_DEM_GEAR_RATIO_STEP_MPV (1)
      | Data Axis: TQ_DEM_KI_DATA_MPV (1/s)
      | Interpolation Method: Linear
  2D_Lookup_Table2 : PTC_MBDS_LIB/Extras/Lookup Tables/2D_Lookup_Table  ParameterObjectName=TQ_DEM_KD_DATA_MPV  InterpolationMethod=Linear  PTC_MBDS_BlockVersion=5.41  PTC_BlockType=PTC_MBDS_2D_Lookup_Table
      settings: SourceProductName=PACCAR Technical Center MBDS Library
      settings: AttributesFormatString=|
      | Row Axis: TQ_DEM_MASS_STEP_MPV (kg)
      | Column Axis: TQ_DEM_GEAR_RATIO_STEP_MPV (1)
      | Data Axis: TQ_DEM_KD_DATA_MPV (s)
      | Interpolation Method: Linear
  gpid_kp : Outport
  gpid_ki : Outport  Port=2
  gpid_kd : Outport  Port=3
  wires:
  2D_Lookup_Table/1 -> gpid_kp/1
  SPN526_TransActualGearRatio/1 -> 2D_Lookup_Table/2, 2D_Lookup_Table2/2, 2D_Lookup_Table1/2
  SPN1760_GrossCombinationVehicleWeight/1 -> 2D_Lookup_Table/1, 2D_Lookup_Table2/1, 2D_Lookup_Table1/1
  2D_Lookup_Table1/1 -> gpid_ki/1
  2D_Lookup_Table2/1 -> gpid_kd/1

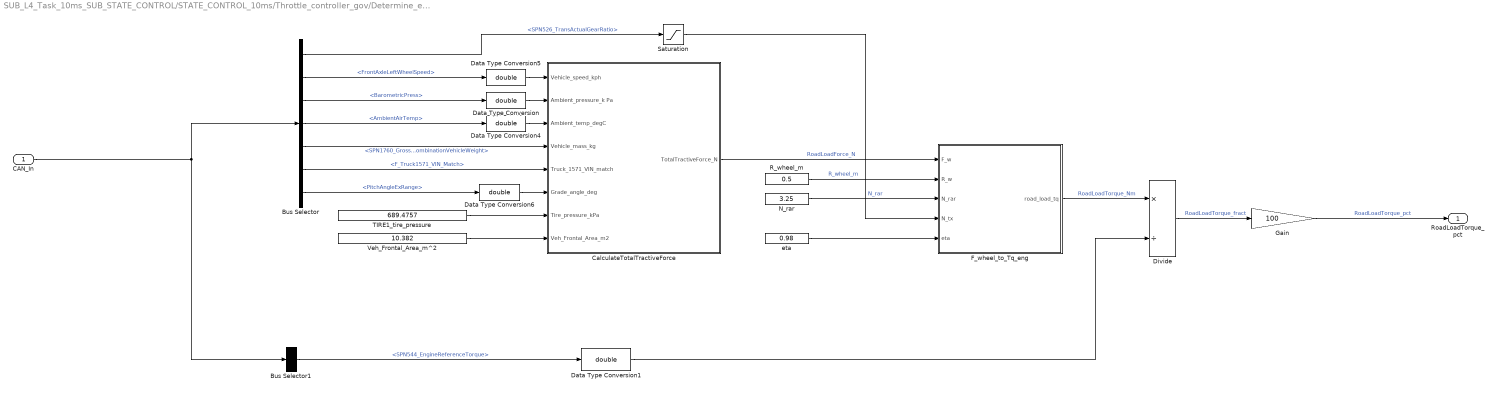
== system SUB_L4_Task_10ms_SUB_STATE_CONTROL/STATE_CONTROL_10ms/Throttle_controller_gov/Determine_engine_torque_and_losses/CalculateRoadLoadTorque ==
  CAN_In : Inport
  Bus Selector : BusSelector  OutputSignals=CAN.ETC2_03.SPN526_TransActualGearRatio,CAN.HRW_0B.FrontAxleLeftWheelSpeed,CAN.AMB_00.BarometricPress,CAN.AMB_00.AmbientAirTemp,CAN.CVW_0B.SPN1760_GrossCombinationVehicleWeight,CAN.VI_00.F_Truck1571_VIN_Match,CAN.SSI2_03.PitchAngleExRange
  Bus Selector1 : BusSelector  OutputSignals=CAN.EC1_00.SPN544_EngineReferenceTorque
  CalculateTotalTractiveForce : Subsystem
  Data Type Conversion{,1,4..6} (5 alike) : DataTypeConversion  OutDataTypeStr=double
      Data Type Conversion settings: AttributesFormatString=%<OutDataTypeStr>
      Data Type Conversion4 settings: AttributesFormatString=%<OutDataTypeStr>
      Data Type Conversion5 settings: AttributesFormatString=%<OutDataTypeStr>
      Data Type Conversion6 settings: AttributesFormatString=%<OutDataTypeStr>
  Divide : Product  Inputs=*/  InputSameDT=on
  F_wheel_to_Tq_eng : MATLAB Function  TreatAsAtomicUnit=on
  Gain : Gain  Gain=100
  N_rar : Constant  Value=3.25
  R_wheel_m : Constant  Value=0.5
  Saturation : Saturate  UpperLimit=20  LowerLimit=0.1
  TIRE1_tire_pressure : Constant  Value=689.4757
  Veh_Frontal_Area_m^2 : Constant  Value=10.382
  eta : Constant  Value=0.98
  RoadLoadTorque_pct : Outport
  wires:
  Data Type Conversion1/1 -> Divide/2
  Divide/1 -> Gain/1  "RoadLoadTorque_fract"
  CalculateTotalTractiveForce/1(TotalTractiveForce_N) -> F_wheel_to_Tq_eng/1(F_w)  "RoadLoadForce_N"
  Bus Selector/6 -> CalculateTotalTractiveForce/5(Truck_1571_VIN_match)  "<F_Truck1571_VIN_Match>"
  Bus Selector/3 -> Data Type Conversion/1  "<BarometricPress>"
  TIRE1_tire_pressure/1 -> CalculateTotalTractiveForce/7(Tire_pressure_kPa)
  Veh_Frontal_Area_m^2/1 -> CalculateTotalTractiveForce/8(Veh_Frontal_Area_m2)
  Data Type Conversion/1 -> CalculateTotalTractiveForce/2(Ambient_pressure_k Pa)
  Bus Selector/7 -> Data Type Conversion6/1  "<PitchAngleExRange>"
  Bus Selector/2 -> Data Type Conversion5/1  "<FrontAxleLeftWheelSpeed>"
  Data Type Conversion4/1 -> CalculateTotalTractiveForce/3(Ambient_temp_degC)
  Bus Selector/4 -> Data Type Conversion4/1  "<AmbientAirTemp>"
  Data Type Conversion5/1 -> CalculateTotalTractiveForce/1(Vehicle_speed_kph)
  CAN_In/1 -> Bus Selector1/1, Bus Selector/1
  Bus Selector/5 -> CalculateTotalTractiveForce/4(Vehicle_mass_kg)  "<SPN1760_GrossCombinationVehicleWeight>"
  F_wheel_to_Tq_eng/1(road_load_tq) -> Divide/1  "RoadLoadTorque_Nm"
  R_wheel_m/1 -> F_wheel_to_Tq_eng/2(R_w)  "R_wheel_m"
  eta/1 -> F_wheel_to_Tq_eng/5(eta)
  N_rar/1 -> F_wheel_to_Tq_eng/3(N_rar)  "N_rar"
  Saturation/1 -> F_wheel_to_Tq_eng/4(N_tx)
  Bus Selector/1 -> Saturation/1  "<SPN526_TransActualGearRatio>"
  Gain/1 -> RoadLoadTorque_pct/1  "RoadLoadTorque_pct"
  Bus Selector1/1 -> Data Type Conversion1/1  "<SPN544_EngineReferenceTorque>"
  Data Type Conversion6/1 -> CalculateTotalTractiveForce/6(Grade_angle_deg)

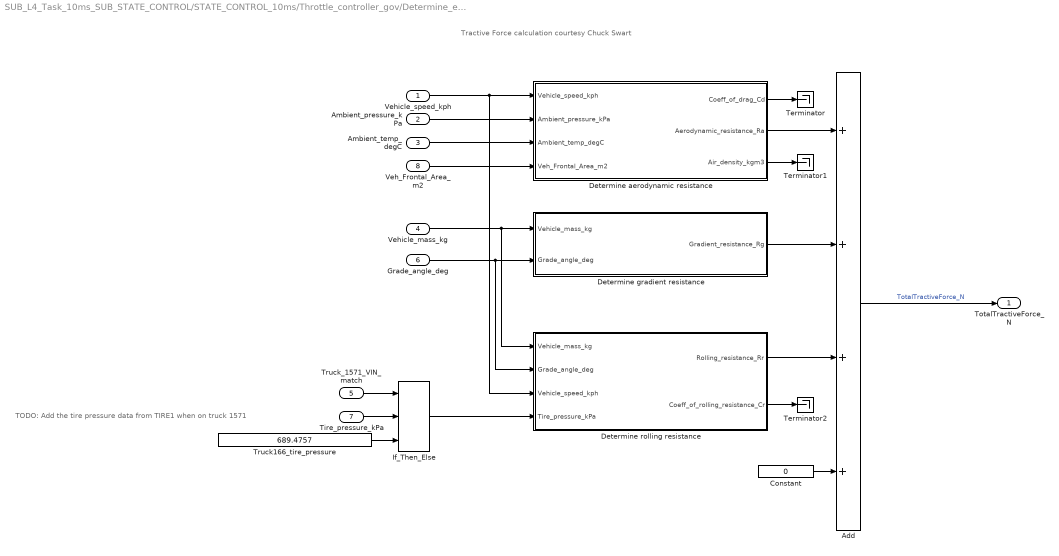
== system SUB_L4_Task_10ms_SUB_STATE_CONTROL/STATE_CONTROL_10ms/Throttle_controller_gov/Determine_engine_torque_and_losses/CalculateRoadLoadTorque/CalculateTotalTractiveForce ==
  note: TODO: Add the tire pressure data from TIRE1 when on truck 1571
  note: Tractive Force calculation courtesy Chuck Swart
  Vehicle_speed_kph : Inport
  Ambient_pressure_k Pa : Inport  Port=2
  Ambient_temp_degC : Inport  Port=3
  Vehicle_mass_kg : Inport  Port=4
  Truck_1571_VIN_match : Inport  Port=5
  Grade_angle_deg : Inport  Port=6
  Tire_pressure_kPa : Inport  Port=7
  Veh_Frontal_Area_m2 : Inport  Port=8
  Add : Sum  Inputs=++++  InputSameDT=on
  Constant : Constant  Value=0
  Determine aerodynamic resistance : Subsystem
  Determine gradient resistance : Subsystem
  Determine rolling resistance : Subsystem
  If_Then_Else : EmE_MBD_Blockset/Signal Routing/If_Then_Else
      settings: SourceProductName=PACCAR EmE MBD Blockset
  Terminator : Terminator
  Terminator1 : Terminator
  Terminator2 : Terminator
  Truck166_tire_pressure : Constant  Value=689.4757
  TotalTractiveForce_N : Outport
  wires:
  If_Then_Else/1 -> Determine rolling resistance/4(Tire_pressure_kPa)
  Determine rolling resistance/2(Coeff_of_rolling_resistance_Cr) -> Terminator2/1
  Determine rolling resistance/1(Rolling_resistance_Rr) -> Add/3
  Ambient_pressure_k Pa/1 -> Determine aerodynamic resistance/2(Ambient_pressure_kPa)
  Add/1 -> TotalTractiveForce_N/1  "TotalTractiveForce_N"
  Vehicle_speed_kph/1 -> Determine rolling resistance/3(Vehicle_speed_kph), Determine aerodynamic resistance/1(Vehicle_speed_kph)
  Ambient_temp_degC/1 -> Determine aerodynamic resistance/3(Ambient_temp_degC)
  Determine aerodynamic resistance/1(Coeff_of_drag_Cd) -> Terminator/1
  Veh_Frontal_Area_m2/1 -> Determine aerodynamic resistance/4(Veh_Frontal_Area_m2)
  Constant/1 -> Add/4
  Vehicle_mass_kg/1 -> Determine rolling resistance/1(Vehicle_mass_kg), Determine gradient resistance/1(Vehicle_mass_kg)
  Grade_angle_deg/1 -> Determine rolling resistance/2(Grade_angle_deg), Determine gradient resistance/2(Grade_angle_deg)
  Determine gradient resistance/1(Gradient_resistance_Rg) -> Add/2
  Determine aerodynamic resistance/3(Air_density_kgm3) -> Terminator1/1
  Determine aerodynamic resistance/2(Aerodynamic_resistance_Ra) -> Add/1
  Tire_pressure_kPa/1 -> If_Then_Else/2
  Truck166_tire_pressure/1 -> If_Then_Else/3
  Truck_1571_VIN_match/1 -> If_Then_Else/1

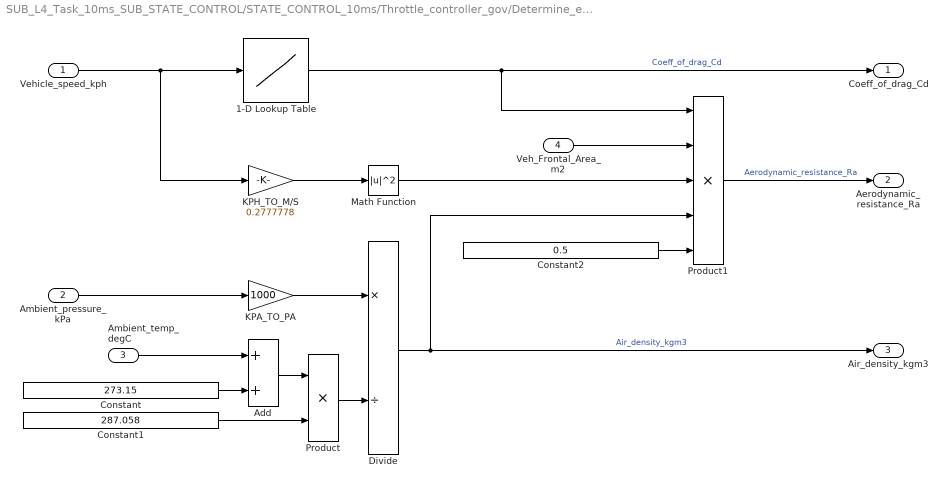
== system SUB_L4_Task_10ms_SUB_STATE_CONTROL/STATE_CONTROL_10ms/Throttle_controller_gov/Determine_engine_torque_and_losses/CalculateRoadLoadTorque/CalculateTotalTractiveForce/Determine aerodynamic resistance ==
  Vehicle_speed_kph : Inport
  Ambient_pressure_kPa : Inport  Port=2
  Ambient_temp_degC : Inport  Port=3
  Veh_Frontal_Area_m2 : Inport  Port=4
  1-D Lookup Table : Lookup_n-D  NumberOfTableDimensions=1  BreakpointsForDimension1=[0 1 200]  Table=[0 0.5779 0.5779]  TableDataTypeStr=Inherit: Inherit from 'Table data'  ExtrapMethod=Clip  UseLastTableValue=on  OutDataTypeStr=Inherit: Inherit from 'Table data'  InputSameDT=on
      settings: AttributesFormatString=|
      | X: %<BreakpointsForDimension1>
      | Y: %<Table>
  Add : Sum  InputSameDT=on
  Constant : Constant  Value=273.15
  Constant1 : Constant  Value=287.058
  Constant2 : Constant  Value=0.5
  Divide : Product  Inputs=*/  InputSameDT=on
  KPA_TO_PA : Gain  Gain=1000  OutDataTypeStr=double
  KPH_TO_M/S : Gain  Gain=0.2777778  OutDataTypeStr=double
  Math Function : Math  Operator=magnitude^2  SaturateOnIntegerOverflow=on
  Product : Product  InputSameDT=on
  Product1 : Product  Inputs=5  InputSameDT=on
  Coeff_of_drag_Cd : Outport
  Aerodynamic_resistance_Ra : Outport  Port=2
  Air_density_kgm3 : Outport  Port=3
  wires:
  KPA_TO_PA/1 -> Divide/1
  Ambient_temp_degC/1 -> Add/1
  Constant/1 -> Add/2
  Add/1 -> Product/1
  Constant1/1 -> Product/2
  Product/1 -> Divide/2
  Constant2/1 -> Product1/5
  Divide/1 -> Product1/4, Air_density_kgm3/1  "Air_density_kgm3"
  Veh_Frontal_Area_m2/1 -> Product1/2
  Math Function/1 -> Product1/3
  1-D Lookup Table/1 -> Coeff_of_drag_Cd/1, Product1/1  "Coeff_of_drag_Cd"
  Product1/1 -> Aerodynamic_resistance_Ra/1  "Aerodynamic_resistance_Ra"
  Vehicle_speed_kph/1 -> KPH_TO_M/S/1, 1-D Lookup Table/1
  Ambient_pressure_kPa/1 -> KPA_TO_PA/1
  KPH_TO_M/S/1 -> Math Function/1

== system SUB_L4_Task_10ms_SUB_STATE_CONTROL/STATE_CONTROL_10ms/Throttle_controller_gov/Determine_engine_torque_and_losses/CalculateRoadLoadTorque/CalculateTotalTractiveForce/Determine gradient resistance ==
  Vehicle_mass_kg : Inport
  Grade_angle_deg : Inport  Port=2
  Constant1 : Constant  Value=9.807
  Constant2 : Constant  Value=pi
  Constant3 : Constant  Value=180
  Divide : Product  Inputs=**/  InputSameDT=on
  Product1 : Product  Inputs=3  InputSameDT=on
  Trigonometric Function : Trigonometry
  Gradient_resistance_Rg : Outport
  wires:
  Constant1/1 -> Product1/3
  Vehicle_mass_kg/1 -> Product1/1
  Trigonometric Function/1 -> Product1/2
  Grade_angle_deg/1 -> Divide/1
  Constant3/1 -> Divide/3
  Constant2/1 -> Divide/2
  Divide/1 -> Trigonometric Function/1  "grade_angle_radians"
  Product1/1 -> Gradient_resistance_Rg/1  "Gradient_resistance_Rg"

== system SUB_L4_Task_10ms_SUB_STATE_CONTROL/STATE_CONTROL_10ms/Throttle_controller_gov/Determine_engine_torque_and_losses/CalculateRoadLoadTorque/CalculateTotalTractiveForce/Determine rolling resistance ==
  Vehicle_mass_kg : Inport
  Grade_angle_deg : Inport  Port=2
  Vehicle_speed_kph : Inport  Port=3
  Tire_pressure_kPa : Inport  Port=4
  Constant3 : Constant  Value=9.807
  Constant4 : Constant  Value=pi
  Constant5 : Constant  Value=180
  Determine coefficient of rolling resistance : Subsystem
  Divide1 : Product  Inputs=**/  InputSameDT=on
  Product2 : Product  Inputs=4  InputSameDT=on
  Trigonometric Function : Trigonometry  Operator=cos
  Rolling_resistance_Rr : Outport
  Coeff_of_rolling_resistance_Cr : Outport  Port=2
  wires:
  Constant3/1 -> Product2/4
  Trigonometric Function/1 -> Product2/3
  Constant5/1 -> Divide1/3
  Constant4/1 -> Divide1/2
  Divide1/1 -> Trigonometric Function/1  "grade_angle_radians"
  Vehicle_mass_kg/1 -> Product2/2
  Grade_angle_deg/1 -> Divide1/1
  Product2/1 -> Rolling_resistance_Rr/1  "Rolling_resistance_Rr"
  Vehicle_speed_kph/1 -> Determine coefficient of rolling resistance/1(Vehicle_speed_kph)
  Tire_pressure_kPa/1 -> Determine coefficient of rolling resistance/2(Tire_pressure_kPa)
  Determine coefficient of rolling resistance/1(Coeff_of_rolling_resistance_Cr) -> Coeff_of_rolling_resistance_Cr/1, Product2/1

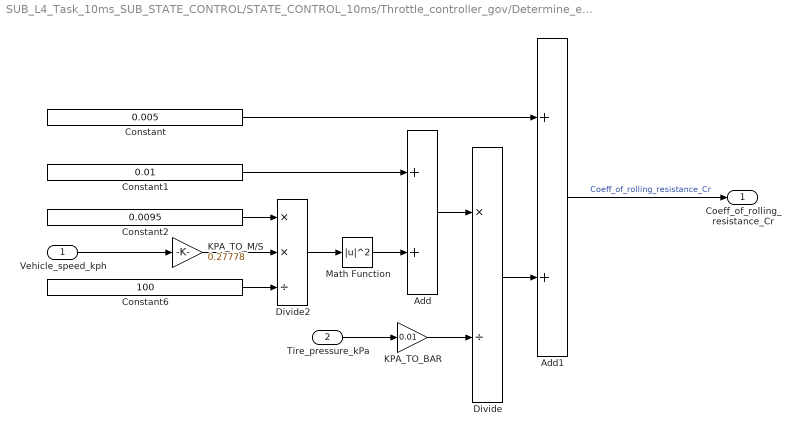
== system SUB_L4_Task_10ms_SUB_STATE_CONTROL/STATE_CONTROL_10ms/Throttle_controller_gov/Determine_engine_torque_and_losses/CalculateRoadLoadTorque/CalculateTotalTractiveForce/Determine rolling resistance/Determine coefficient of rolling resistance ==
  Vehicle_speed_kph : Inport
  Tire_pressure_kPa : Inport  Port=2
  Add : Sum  InputSameDT=on
  Add1 : Sum  InputSameDT=on
  Constant : Constant  Value=0.005
  Constant1 : Constant  Value=0.01
  Constant2 : Constant  Value=0.0095
  Constant6 : Constant  Value=100
  Divide : Product  Inputs=*/  InputSameDT=on
  Divide2 : Product  Inputs=**/  InputSameDT=on
  KPA_TO_BAR : Gain  Gain=0.01
  KPA_TO_M/S : Gain  Gain=0.27778
  Math Function : Math  Operator=magnitude^2  SaturateOnIntegerOverflow=on
  Coeff_of_rolling_resistance_Cr : Outport
  wires:
  Constant1/1 -> Add/1
  Constant6/1 -> Divide2/3
  Constant2/1 -> Divide2/1
  Constant/1 -> Add1/1
  Add/1 -> Divide/1
  Add1/1 -> Coeff_of_rolling_resistance_Cr/1  "Coeff_of_rolling_resistance_Cr"
  Math Function/1 -> Add/2
  Divide2/1 -> Math Function/1
  KPA_TO_BAR/1 -> Divide/2
  Divide/1 -> Add1/2
  Tire_pressure_kPa/1 -> KPA_TO_BAR/1
  Vehicle_speed_kph/1 -> KPA_TO_M/S/1
  KPA_TO_M/S/1 -> Divide2/2

== stateflow chart SUB_L4_Task_10ms_SUB_STATE_CONTROL/STATE_CONTROL_10ms/Relay_control/Relay_control_state_machine ==
  state INITIAL
    en:
    F_Ignition_relay_command = false;
    F_Inverter_relay_command = false;
    F_MABX_relay_command = false;
    F_Sensor_relay_command = false;
    IGN_RELAY_ON_DELAY_SECS_APV = On_delay_bus(1);
    INVERTER_RELAY_ON_DELAY_SECS_APV = On_delay_bus(2);
    MABX_RELAY_ON_DELAY_SECS_APV = On_delay_bus(3);
    SENSOR_RELAY_ON_DELAY_SECS_APV = On_delay_bus(4);
    IGN_RELAY_OFF_DELAY_SECS_APV = Off_delay_bus(1);
    INVERTER_RELAY_OFF_DELAY_SECS_APV = Off_delay_bus(2);
    MABX_RELAY_OFF_DELAY_SECS_APV = Off_delay_bus(3);
    SENSOR_RELAY_OFF_DELAY_SECS_APV = Off_delay_bus(4);
  state POWER_UP_ROUTINE
    state WAIT
    state MABX_RELAY_LATCH
      en:
      F_MABX_relay_command = true;
    state SENSOR_RELAY_LATCH
      en:
      F_Sensor_relay_command = true;
    state INV_RELAY_LATCH
      en:
      F_Inverter_relay_command = true;
    state IGN_RELAY_LATCH
      en:
      F_Ignition_relay_command = true;
    (default) -> POWER_UP_ROUTINE.WAIT
    POWER_UP_ROUTINE.WAIT -> MABX_RELAY_LATCH : after(MABX_RELAY_ON_DELAY_SECS_APV,sec)
    MABX_RELAY_LATCH -> SENSOR_RELAY_LATCH : after(SENSOR_RELAY_ON_DELAY_SECS_APV,sec)
    SENSOR_RELAY_LATCH -> INV_RELAY_LATCH : after(INVERTER_RELAY_ON_DELAY_SECS_APV,sec)
    INV_RELAY_LATCH -> IGN_RELAY_LATCH : after(IGN_RELAY_ON_DELAY_SECS_APV,sec)
  state POWER_DOWN_ROUTINE
    state WAIT
    state IGN_RELAY_UNLATCH
      en:
      F_Ignition_relay_command = false;
    state INV_RELAY_UNLATCH
      en:
      F_Inverter_relay_command = false;
    state SENSOR_RELAY_UNLATCH
      en:
      F_Sensor_relay_command = false;
    state MABX_RELAY_UNLATCH
      en:
      F_MABX_relay_command = false;
    (default) -> POWER_DOWN_ROUTINE.WAIT
    POWER_DOWN_ROUTINE.WAIT -> IGN_RELAY_UNLATCH : after(IGN_RELAY_OFF_DELAY_SECS_APV,sec)
    IGN_RELAY_UNLATCH -> INV_RELAY_UNLATCH : after(INVERTER_RELAY_OFF_DELAY_SECS_APV,sec)
    INV_RELAY_UNLATCH -> SENSOR_RELAY_UNLATCH : after(SENSOR_RELAY_OFF_DELAY_SECS_APV,sec)
    SENSOR_RELAY_UNLATCH -> MABX_RELAY_UNLATCH : after(MABX_RELAY_OFF_DELAY_SECS_APV,sec)
  (default) -> INITIAL
  (junction 44) -> INITIAL
  (junction 43) -> (junction 44)
  INITIAL -> POWER_UP_ROUTINE : [F_Ignition_sw_on]
  POWER_UP_ROUTINE -> POWER_DOWN_ROUTINE : [~F_Ignition_sw_on && ...
      | F_Ignition_sw_off_conditions_met]
  MABX_RELAY_UNLATCH -> (junction 42)
  (junction 42) -> (junction 43)
  data: F_Ignition_sw_on input; F_Ignition_sw_off_conditions_met input; On_delay_bus input; Off_delay_bus input; F_Ignition_relay_command output; F_Inverter_relay_command output; F_MABX_relay_command output; F_Sensor_relay_command output; INVERTER_RELAY_ON_DELAY_SECS_APV local; SENSOR_RELAY_ON_DELAY_SECS_APV local; IGN_RELAY_OFF_DELAY_SECS_APV local; INVERTER_RELAY_OFF_DELAY_SECS_APV local; MABX_RELAY_ON_DELAY_SECS_APV local; MABX_RELAY_OFF_DELAY_SECS_APV local; SENSOR_RELAY_OFF_DELAY_SECS_APV local; IGN_RELAY_ON_DELAY_SECS_APV local

== matlab function SUB_L4_Task_10ms_SUB_STATE_CONTROL/STATE_CONTROL_10ms/Throttle_controller_gov/Determine_engine_torque_and_losses/CalculateRoadLoadTorque/F_wheel_to_Tq_eng ==
  data: F_w input; road_load_tq output; R_w input; N_rar input; N_tx input; eta input
function road_load_tq = F_wheel_to_Tq_eng(F_w, R_w, N_rar, N_tx, eta)
%#codegen    
    road_load_tq = F_w * R_w * 1/N_rar * 1/N_tx * 1/eta;

== stateflow chart SUB_L4_Task_10ms_SUB_STATE_CONTROL/STATE_CONTROL_10ms/Chart ==
  state Init
    entry: CtrlState=ENUM_AUTO_CTRL_STATE_T.INIT;
  state OperatorDisabled
    entry: CtrlState=ENUM_AUTO_CTRL_STATE_T.OPERATOR_DISABLED;
  state OperatorEnabled
    entry: CtrlState=ENUM_AUTO_CTRL_STATE_T.AUTO_CTRL_ENABLED;
    state AutoControlEnabled
      state init
        entry: VehCtrlState=ENUM_AUTO_CTRL_VEHICLE_STATE_T.INIT
      (default) -> init
    (default) -> AutoControlEnabled
  (default) -> Init
  Init -> OperatorDisabled : [FAULT_ACTIVE == 0]
  OperatorEnabled -> OperatorDisabled : [OperatorEnableSwitch == 0 || ...
      | FAULT_ACTIVE != 0]
  OperatorDisabled -> OperatorEnabled : [OperatorEnableSwitch == 1]
  data: data local double; OperatorEnableSwitch input boolean; VehicleSpeed_kph input single; OperatorBrakeApplication input uint8; CtrlState output Enum: ENUM_AUTO_CTRL_STATE_T; FAULT_ACTIVE input boolean; VehCtrlState output Enum: ENUM_AUTO_CTRL_VEHICLE_STATE_T =ENUM_AUTO_CTRL_VEHICLE_STATE_T.NOT_AVAILABLE
